simulink model "demo_i"  (R2021a)
settings: Solver=VariableStepAuto  StartTime=0.0  StopTime=0.4  FixedStep=0.001  RelTol=1e-3
PostLoadFcn:
  | , if any(exist('dsrtsu_mdlpostloadfcn', 'file') == [2, 3, 6]), try dsrtsu_mdlpostloadfcn('Execute', bdroot); catch fprintf('Error in PostLoadFcn (dsrtsu_mdlpostloadfcn) for model "%s":\n %s\n', bdroot, lasterr); end, end,
libraries: spsSeriesRLCBranchLib x3, spsCurrentMeasurementLib x2, spsControlledCurrentSourceLib x1, spsControlledVoltageSourceLib x1, spsDiodeLib x1, spsMosfetLib x1, spsVoltageMeasurementLib x1, spspowerguiLib x1, spsPWMGeneratorDCDCLib x1
(part 1 of 3)
Description:
  | Standard RTI1006 template.
  | Supported MATLAB version:  R2019a.
settings Model: Tag=RTI1006  DSRTSU_INTERNAL_RTI_VER=540  DSRTSU_INTERNAL_RTI_TYPE=rti1006  RTICANMMDATA=struct('GeneralSetupData',struct('modelroot','E:\WORK\MigrationScripts','generalsettings',struct('filesettings',struct('destfolder',struct('Name','RTICANMM_FILES','Check',1),'buildfolder',struct('Name','.','Check',1),'AbsDestfolder',struct('Name','E:\WORK\MigrationScripts\RTICANMM_FILES'),'AbsBuildfolder',struct('Name','E:\WORK\MigrationScripts'))),'options',struct('addpaths',1,'rmpaths',1,'addtrcexclusion',logical(1),'cannavigator',struct('checkmonitoring',0),'show_usrtrc',0,'use_usrtrc',0),'advanced',struct('options',ones(1,100)),'MPSetup',{{}},'RTI',struct('Type','RTI1006','Ver','7.12','Date','02-May-2019'),'modelname','','block','untitled'))  DSRTSU_INTERNAL_RTIFPGA=130  Creator=user  LastModifiedBy=86182
settings SolverCC: AlgebraicLoopSolver=TrustRegion
settings DataIOCC: ReturnWorkspaceOutputs=off
settings OptimizationCC: BlockReduction=off  OptimizeBlockIOStorage=off  BufferReuse=off  GlobalBufferReuse=off  ExpressionFolding=off  LocalBlockOutputs=off  OptimizeDataStoreBuffers=off  BusAssignmentInplaceUpdate=off
settings DebuggingCC: PregeneratedLibrarySubsystemCodeDiagnostic=none  SFMachineParentedDataDiag=warning  ArithmeticOperatorsInVariantConditions=warning
settings HardwareCC: ProdBitPerPointer=32  ProdBitPerSizeT=32  ProdBitPerPtrDiffT=32  ProdLargestAtomicInteger=Integer  ProdWordSize=32  ProdHWDeviceType=Custom Processor->Custom  TargetIntDivRoundTo=Zero  TargetEndianess=LittleEndian  TargetHWDeviceType=Custom Processor->Custom
settings SFSimCC: SimUseLocalCustomCode=off  MATLABDynamicMemAlloc=off  CustomCodeUndefinedFunction=UseInterfaceOnly
settings RTWCC: Description=dSPACE DS1006 Hardware Platform  SystemTargetFile=rti1006.tlc  MakeCommand=make_rti  TemplateMakefile=rti1006.tmf  RTWUseLocalCustomCode=off
settings CodeAppCC: StateflowObjectComments=on
settings STFCustomTargetCC: ParMdlRefBuildCompliant=on  MatFileLogging=on  GRTInterface=off  UseToolchainInfoCompliant=off  SystemTargetFile=rti1006.tlc
settings GRTTargetCC: TargetLangStandard=C89/C90 (ANSI)  CompOptLevelCompliant=off  ConcurrentExecutionCompliant=off  CombineOutputUpdateFcns=off  CPPClassGenCompliant=off  UseToolchainInfoCompliant=off
settings ConfigComp: CovMetricSettings=dswe

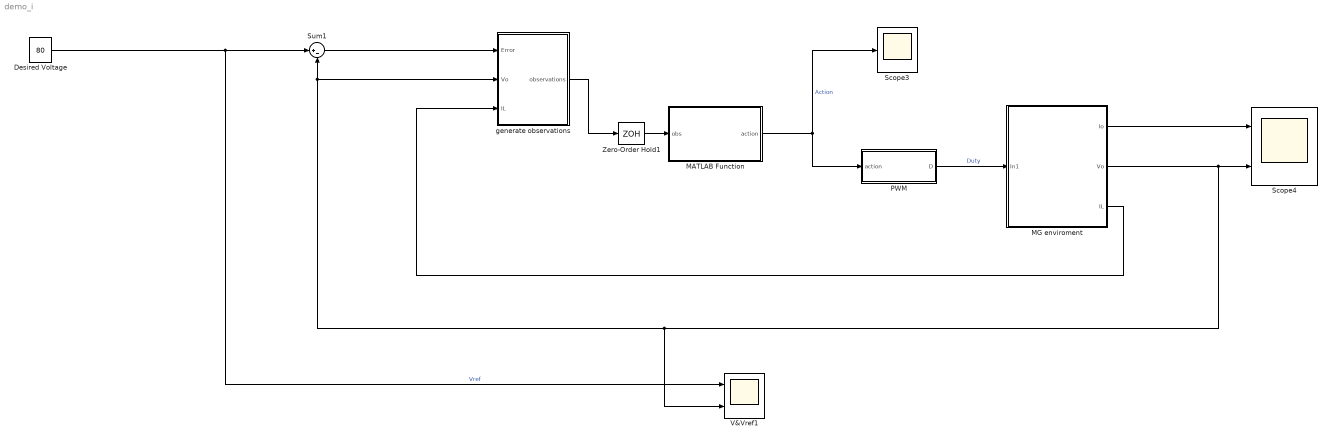
== system demo_i ==
  Desired Voltage : Constant  Value=80
  MATLAB Function : MATLAB Function  TreatAsAtomicUnit=on
  "MG enviroment " : Subsystem
  PWM : Subsystem
  Scope3 : Scope
  Scope4 : Scope  NumInputPorts=2
  Sum1 : Sum  Inputs=|+-  SaturateOnIntegerOverflow=on
  V&Vref1 : Scope  NumInputPorts=2
  Zero-Order Hold1 : ZeroOrderHold  SampleTime=1e-4
  generate observations : Subsystem
  wires:
  Sum1/1 -> generate observations/1(Error)
  Desired Voltage/1 -> V&Vref1/1, Sum1/1  "Vref"
  PWM/1(D) -> "MG enviroment "/1(In1)  "Duty"
  "MG enviroment "/1(Io) -> Scope4/1
  MATLAB Function/1(action) -> Scope3/1, PWM/1(action)  "Action"
  "MG enviroment "/2(Vo) -> Scope4/2, V&Vref1/2, Sum1/2, generate observations/2(Vo)
  "MG enviroment "/3(IL) -> generate observations/3(IL)
  generate observations/1(observations) -> Zero-Order Hold1/1
  Zero-Order Hold1/1 -> MATLAB Function/1(obs)

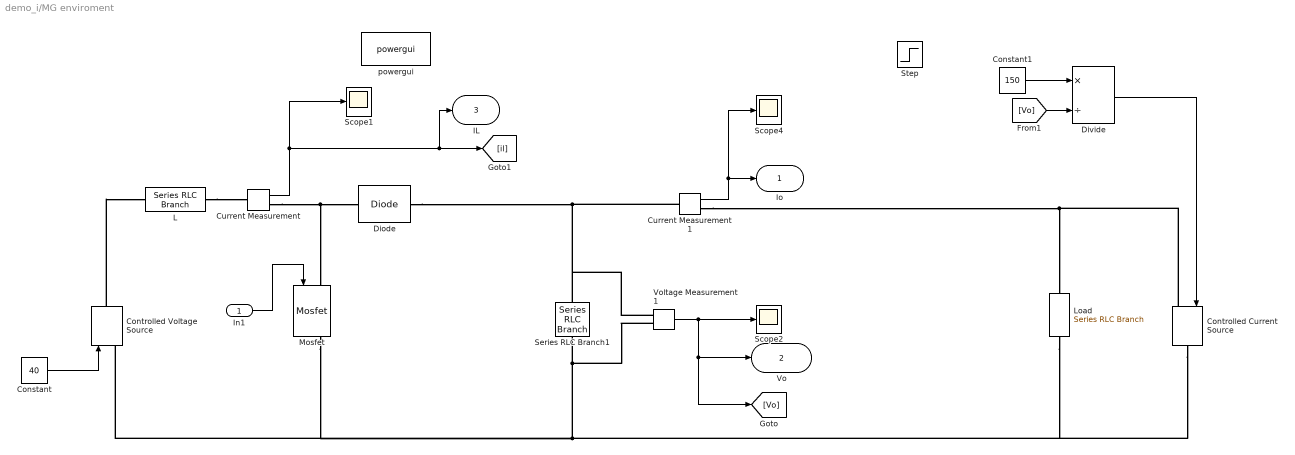
== system demo_i/MG enviroment  ==
  In1 : Inport
  Constant : Constant  Value=40
  Constant1 : Constant  Value=150
  Controlled Current Source : spsControlledCurrentSourceLib/Controlled Current Source  Initialize=on  Source_Type=AC  Amplitude=0  Phase=0  Frequency=0  Measurements=None
  Controlled Voltage Source : spsControlledVoltageSourceLib/Controlled Voltage Source  Initialize=on  Source_Type=DC  Amplitude=50  Phase=0  Frequency=0  Measurements=None
  Current Measurement : spsCurrentMeasurementLib/Current Measurement  PhasorSimulation=off  OutputType=Complex  PSBequivalent=0
  Current Measurement1 : spsCurrentMeasurementLib/Current Measurement  PhasorSimulation=off  OutputType=Complex  PSBequivalent=0
  Diode : spsDiodeLib/Diode  Ron=0.00001  Lon=0  Vf=0  IC=0  UseSnubber=0  Rs=500000  Cs=10e-9  Measurements=off
  Divide : Product  Inputs=*/
  L : spsSeriesRLCBranchLib/Series RLC Branch  LConnTagsString=__new0  RConnTagsString=__new0  BranchType=L  Resistance=0.003  Inductance=0.0068  SetiL0=off  InitialCurrent=2  Capacitance=1e-6  Setx0=off  InitialVoltage=0  Measurements=None
  Load : spsSeriesRLCBranchLib/Series RLC Branch  LConnTagsString=__new0  RConnTagsString=__new0  BranchType=R  Resistance=10000  Inductance=200e-6  SetiL0=off  InitialCurrent=0  Capacitance=400e-6  Setx0=off  InitialVoltage=0  Measurements=None
  Mosfet : spsMosfetLib/Mosfet  Ron=0.01  Lon=0  Rd=0.01  Vfd=0  IC=0  Rs=1e5  Cs=inf  Measurements=on
  Scope1 : Scope
  Scope2 : Scope
  Scope4 : Scope
  Series RLC Branch1 : spsSeriesRLCBranchLib/Series RLC Branch  LConnTagsString=__new0  RConnTagsString=__new0  BranchType=C  Resistance=1e-4  Inductance=200e-6  SetiL0=off  InitialCurrent=0  Capacitance=0.0018  Setx0=on  InitialVoltage=80  Measurements=None
  Step : Step  Time=0.4  Before=150  After=250  SampleTime=0
  Voltage Measurement1 : spsVoltageMeasurementLib/Voltage Measurement  PhasorSimulation=off  OutputType=Complex  PSBequivalent=0
  powergui : spspowerguiLib/powergui  Priority=1  SimulationMode=Continuous  SampleTime=50e-6  frequency=60  Iterations=50  frequencyindice=0  Pbase=100e6  ErrMax=1e-4  UnitsV=kV  UnitsW=MW  buscounter=0  FunctionMessages=off  echomessages=off  EnableUseOfTLC=off  CurrentSourceSwitches=off  DisableSnubberDevices=off  DisableRonSwitches=off  DisableVfSwitches=off  DisplayEquations=off  AutomaticDiscreteSolvers=off  SolverType=Tustin/Backward Euler (TBE)  Interpol=off  ExternalGateDelay=off  methode=off  Ts=100  x0status=blocks  SPID=on  SwTol=0  HookPort=off  NonlinearTolerance=0  nMaxIteration=15  ContinueOnMaxIteration=off  RestoreLinks=warning  ResistiveCurrentMeasurement=off  Frange=[0:2:500]  Ylog=off  Xlog=on  ShowGrid=off  save=off  variable=ZData  structure=0  ZoomFFT=off  StartTime=0.0  cycles=1  DisplayStyle=1  fundamental=60  FreqAxis=off  MaxFrequency=1000  frequencyindicesteady=1  RmsSteady=1  display=off
  Io : Outport  VectorParamsAs1DForOutWhenUnconnected=off
  Vo : Outport  Port=2  VectorParamsAs1DForOutWhenUnconnected=off
  IL : Outport  Port=3
  wires:
  Divide/1 -> Controlled Current Source/1
  In1/1 -> Mosfet/1
  Constant/1 -> Controlled Voltage Source/1
  [Vo] -> Divide/2
  Voltage Measurement1/1 -> [Vo], Vo/1, Scope2/1
  Current Measurement1/1 -> Scope4/1, Io/1
  Current Measurement/1 -> IL/1, [il], Scope1/1
  Constant1/1 -> Divide/1
  connections:
  Diode/RConn1 -- Current Measurement1/LConn1 -- Series RLC Branch1/LConn1 -- Voltage Measurement1/LConn1
  Current Measurement1/RConn1 -- Load/LConn1 -- Controlled Current Source/LConn1
  Voltage Measurement1/LConn2 -- Load/RConn1 -- Controlled Current Source/RConn1 -- Mosfet/RConn1 -- Controlled Voltage Source/LConn1 -- Series RLC Branch1/RConn1
  Current Measurement/RConn1 -- Mosfet/LConn1 -- Diode/LConn1
  L/RConn1 -- Current Measurement/LConn1
  Controlled Voltage Source/RConn1 -- L/LConn1

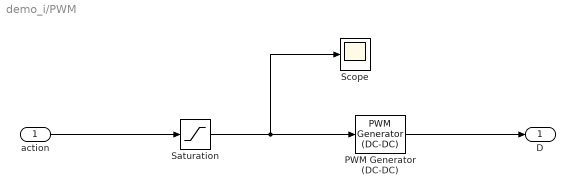
== system demo_i/PWM ==
  action : Inport
  PWM Generator (DC-DC) : spsPWMGeneratorDCDCLib/PWM Generator (DC-DC)  Fsw=10000  Ts=0
  Saturation : Saturate  UpperLimit=0.99  LowerLimit=0.01
  Scope : Scope
  D : Outport  VectorParamsAs1DForOutWhenUnconnected=off
  wires:
  PWM Generator (DC-DC)/1 -> D/1
  Saturation/1 -> Scope/1, PWM Generator (DC-DC)/1
  action/1 -> Saturation/1

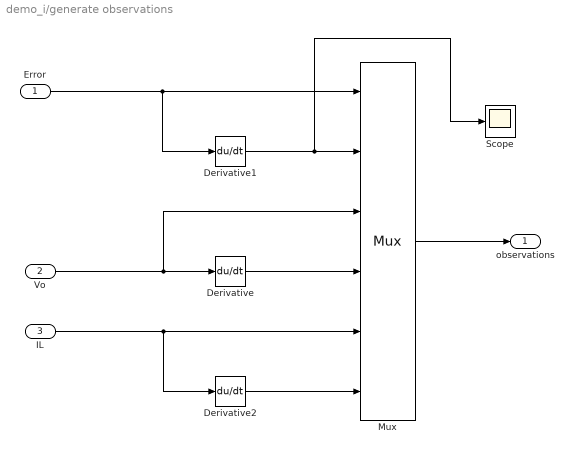
== system demo_i/generate observations ==
  Error : Inport
  Vo : Inport  Port=2
  IL : Inport  Port=3
  Derivative : Derivative
  Derivative1 : Derivative
  Derivative2 : Derivative
  Mux : Mux  Inputs=6
  Scope : Scope
  observations : Outport  VectorParamsAs1DForOutWhenUnconnected=off
  wires:
  Mux/1 -> observations/1
  Derivative1/1 -> Scope/1, Mux/2
  Error/1 -> Derivative1/1, Mux/1
  Derivative/1 -> Mux/4
  Vo/1 -> Mux/3, Derivative/1
  IL/1 -> Derivative2/1, Mux/5
  Derivative2/1 -> Mux/6
